simulink model "main_sim_adapt_Gref_SPPH"  (Simulink 7.2)
settings: Solver=ode2  SolverMode=SingleTasking  StartTime=0.0  StopTime=tsim_max  FixedStep=dtsim  RelTol=1e-3
StopFcn:
  | %mkplt
values from neighbouring files (symbols this model uses):
  assertion_time = inf    [setup_taem_sgs_al.m]
  cosA = cos(rwyAZ_rad)    [setup_taem_sgs_al.m]
  E_rwy = E_origin + (mod(( rwyLLA(2)/constants.r2d - lon_origin )+pi,2*pi)-pi) * constants.earth_radius * cos(lat_origin)    [setup_taem_sgs_al.m]
  eow_boundary = tmp_eow(ix(1))    [setup_taem_sgs_al.m]
  N_rwy = N_origin + (mod(( rwyLLA(1)/constants.r2d - lat_origin )+pi,2*pi)-pi) * constants.earth_radius    [setup_taem_sgs_al.m]
  sinA = sin(rwyAZ_rad)    [setup_taem_sgs_al.m]
  vel = 487.2512    [doit.m]
undefined symbols (not defined in the file or in its folder): accel_cmd, aero_surf_qbar_off, aero_surf_qbar_on, Alon, att_cmd_select, att_trim_IC, att_type, att_type_numbers, B1, bb_ellipsoid, bb_params, Blon, C, CA, chi_trim_IC, Clon, command_time, compute_all_rate_cols, compute_all_vel_cols, constants, da_trim_IC, dc_L2W_IC, de_trim_IC, DiscIntNeverNeededParam, dr_trim_IC, dtsim, DZkx, DZtheta, E_trim_IC, Ed_cmd, Ed_trim_IC, fc, flag_uad, full_surf_llim, full_surf_ulim, gain_set, gain_var_struct, gam_cmd_descent, gam_cmd_preflare, gamdot_cmd_descent, gamdot_cmd_flare, gamdot_cmd_preflare, gamma_trim_IC, Gamtheta, Gamx, h_trim_IC, hd_cmd, hd_trim_IC, ideal_vel_Kb, in_exsig_vecin, in_exsig_vecout, invCB, Kb, Kxhat0, Kxnom, Kxstar, lonxm0, MACH, MACH_att_fb, MACH_att_int_IC ... (+77)
libraries: simulink x36, utility_lib x36, mach_lib x24, model_lib x15, simulink_need_slupdate x8, models x6
(part 2 of 7)

== system main_sim_adapt_Gref_SPPH/claw_main/set scoped signals ==
  signal_bus : Inport  OutDataType=sfix(16)  OutScaling=2^0
  Bus Selector3 : BusSelector  OutputSignals=y_meas.h_geodetic,mode_sw.use_held_aero_obac_sw,y_meas.w_est,y_meas.NEh_dot,mode_sw.att_type,u_est,engines
  Gain1 : Gain  Orientation=left  Gain=use_variable_mass  ParameterDataType=sfix(16)  ParameterScaling=2^0  OutDataType=sfix(16)  OutScaling=2^0
  hold altitude : model_lib/hold input  SystemSampleTime=-1
  mass : DiscreteIntegrator  gainval=1  InitialCondition=MACH_mass_IC  SampleTime=-1  OutDataType=sfix(16)  OutScaling=2^0  ICPrevOutput=DiscIntNeverNeededParam  ICPrevScaledInput=DiscIntNeverNeededParam
  set scoped bus : model_lib/set scoped bus  SystemSampleTime=-1  vehicle_params=obac_params
  set scoped signals : model_lib/set scoped signals  SystemSampleTime=-1
  scoped_bus : Outport  OutDataType=sfix(16)  OutScaling=2^0
  wires:
  signal_bus/1 -> Bus Selector3/1
  Gain1/1 -> mass/1
  Bus Selector3/1 -> hold altitude/1  "<h_geodetic>"
  set scoped bus/2 -> Gain1/1
  set scoped bus/1 -> set scoped signals/1, scoped_bus/1
  mass/1 -> set scoped bus/7
  Bus Selector3/2 -> hold altitude/2  "<use_held_aero_obac_sw>"
  hold altitude/1 -> set scoped bus/1
  Bus Selector3/3 -> set scoped bus/2  "<w_est>"
  Bus Selector3/4 -> set scoped bus/3  "<NEh_dot>"
  Bus Selector3/5 -> set scoped bus/4  "<att_type>"
  Bus Selector3/6 -> set scoped bus/5  "<u_est>"
  Bus Selector3/7 -> set scoped bus/6  "<engines>"

== system main_sim_adapt_Gref_SPPH/claw_main/state est ==
  u_old : Inport  OutDataType=sfix(16)  OutScaling=2^0
  sensors : Inport  Port=2  OutDataType=sfix(16)  OutScaling=2^0
  signal_bus : Inport  Port=3  OutDataType=sfix(16)  OutScaling=2^0
  Bus Creator : BusCreator  Inputs=12
  Bus Creator1 : BusCreator  Inputs=6
  Bus Selector : BusSelector  OutputSignals=mode_sw.reset_pos_sw,mode_sw.nav_enable_sw,mode_sw.wind_est_sw
  Bus Selector1 : BusSelector  OutputSignals=nav_ok,pqr,NED_dot,latlonh,e
  Bus Selector2 : BusSelector  OutputSignals=aero_env.Mach,aero_env.vel,aero_env.alpha,aero_env.beta,aero_env.uvw_rw,aero_env.qbar
  Bus Selector3 : BusSelector  OutputSignals=u_meas,seeker,accels_cg
  Logical Operator : Logic  AllPortsSameDT=off  OutDataTypeMode=boolean  OutDataTypeStr=boolean
  beta_360 : Fcn  Expr=atan2(u(2),u(1))
  cl model : models/gtm-obac  SystemSampleTime=-1
  process inputs : Subsystem
  process sensors : Subsystem
  wind estimator : Subsystem
  y_meas : Outport  OutDataType=sfix(16)  OutScaling=2^0
  x_est : Outport  Port=2  OutDataType=sfix(16)  OutScaling=2^0
  xdot_est : Outport  Port=3  OutDataType=sfix(16)  OutScaling=2^0
  u_est : Outport  Port=4  OutDataType=sfix(16)  OutScaling=2^0
  aero_env_est : Outport  Port=5  OutDataType=sfix(16)  OutScaling=2^0
  w_est_debug : Outport  Port=6  OutDataType=sfix(16)  OutScaling=2^0
  wires:
  sensors/1 -> Bus Selector3/1, process inputs/2(sensors), wind estimator/3(sensors), Bus Selector1/1
  wind estimator/1(w_est) -> cl model/3, Bus Creator/12  "w_est"
  process sensors/8(dircos) -> wind estimator/1(dircos), Bus Creator/11  "dircos"
  cl model/1 -> xdot_est/1
  process sensors/9(x_est) -> cl model/1, wind estimator/2(x), x_est/1
  signal_bus/1 -> Bus Selector/1
  Bus Selector/1 -> process sensors/1(reset_pos)  "<reset_pos_sw>"
  Bus Selector/3 -> wind estimator/5(wind_est_sw)  "<wind_est_sw>"
  process inputs/1(u_est) -> u_est/1, cl model/2, wind estimator/4(u)
  Bus Selector1/2 -> process sensors/3(pqr)  "<pqr>"
  Bus Selector1/3 -> process sensors/4(NED_dot)  "<NED_dot>"
  Bus Selector1/4 -> process sensors/5(latlonh)  "<latlonh>"
  Bus Selector1/5 -> process sensors/6(e)  "<e>"
  process sensors/2(h_geodetic) -> Bus Creator/5  "h_geodetic"
  process sensors/3(NEh_nav) -> Bus Creator/6  "NEh_nav"
  process sensors/4(nav_valid) -> Bus Creator/7  "nav_valid"
  process sensors/5(NEh_dot) -> Bus Creator/8  "NEh_dot"
  process sensors/1(vehicle_origin) -> Bus Creator/4  "vehicle_origin"
  process sensors/7(cvc_origin) -> Bus Creator/10  "cvc_origin"
  u_old/1 -> process inputs/1(u_old)
  wind estimator/2(w_est_debug) -> w_est_debug/1
  cl model/2 -> Bus Selector2/1
  Bus Creator1/1 -> aero_env_est/1
  Logical Operator/1 -> process sensors/2(nav_ok)
  Bus Selector1/1 -> Logical Operator/2  "<nav_ok>"
  Bus Selector/2 -> Logical Operator/1  "<nav_enable_sw>"
  Bus Selector2/5 -> beta_360/1  "<uvw_rw>"
  process sensors/6(dc_fltpath) -> Bus Creator/9  "dc_fltpath"
  beta_360/1 -> Bus Creator1/5  "beta_360"
  Bus Selector2/1 -> Bus Creator1/1  "<Mach>"
  Bus Selector2/2 -> Bus Creator1/2  "<vel>"
  Bus Selector2/3 -> Bus Creator1/3  "<alpha>"
  Bus Selector2/4 -> Bus Creator1/4  "<beta>"
  Bus Selector2/6 -> Bus Creator1/6  "<qbar>"
  Bus Selector3/1 -> Bus Creator/1  "<u_meas>"
  Bus Selector3/2 -> Bus Creator/2  "<seeker>"
  Bus Selector3/3 -> Bus Creator/3  "<accels_cg>"
  Bus Creator/1 -> y_meas/1

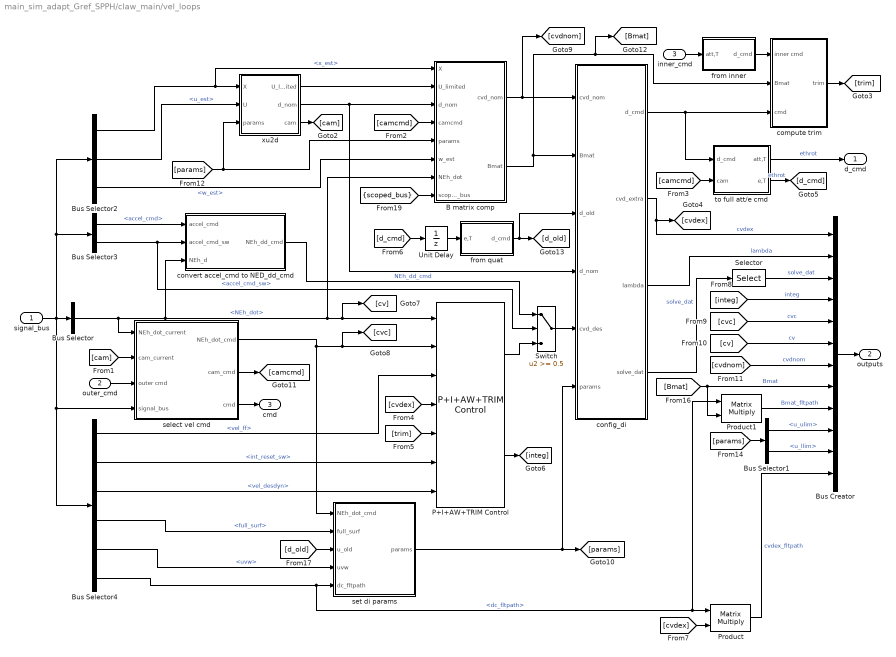
== system main_sim_adapt_Gref_SPPH/claw_main/vel_loops ==
  signal_bus : Inport  OutDataType=sfix(16)  OutScaling=2^0
  outer_cmd : Inport  Port=2  OutDataType=sfix(16)  OutScaling=2^0
  inner_cmd : Inport  Port=3  OutDataType=sfix(16)  OutScaling=2^0
  B matrix comp : Subsystem
  Bus Creator : BusCreator  Inputs=12
  Bus Selector : BusSelector  OutputSignals=y_meas.NEh_dot
  Bus Selector1 : BusSelector  OutputSignals=u_ulim,u_llim
  Bus Selector2 : BusSelector  OutputSignals=x_est,u_est,y_meas.w_est
  Bus Selector3 : BusSelector  OutputSignals=control_params.accel_cmd,control_params.accel_cmd_sw
  Bus Selector4 : BusSelector  OutputSignals=feed_forward.vel_ff,mode_sw.int_reset_sw,control_params.vel_desdyn,full_surf,x_est.uvw,y_meas.dc_fltpath
  P+I+AW+TRIM Control : mach_lib/P+I+AW+TRIM Control  SystemSampleTime=-1
  Product : Product  Multiplication=Matrix(*)  OutDataType=sfix(16)  OutScaling=2^0  RndMeth=Zero
  Product1 : Product  Multiplication=Matrix(*)  OutDataType=sfix(16)  OutScaling=2^0  RndMeth=Zero
  Selector : Selector  NumberOfDimensions=2  InputPortWidth=MACH.num_u  IndexOptions=Index vector (dialog),Index vector (dialog)  Indices=1:9,1:2  OutputSizes=1
  Switch : Switch  Threshold=0.5
  Unit Delay : UnitDelay  X0=MACH_vel_uold_IC  SampleTime=-1
  compute trim : Subsystem
  config_di : Subsystem  BlockChoice=di_smn  mask{num_cv=MACH.vel_num_cv, num_u=MACH.vel_num_u, wght_cv_type=MACH.vel_wght_cv_type}
      link override di_smn/config_smn/smn_sfunc: sfunc_name=MACH.smn_sfunc_name
      link override di_smn/config_smn/smn_sfunc/S-Function: FunctionName=smn_sfunc_gam_mpass_epsposdef
      settings: AttributesFormatString=%<BlockChoice>  TemplateBlock=mach_lib/config_di  MemberBlocks=di_pseudoinv,di_smn
  convert accel_cmd to NED_dd_cmd : Subsystem  TreatAsAtomicUnit=on
  from inner : Subsystem
  from quat : Subsystem
  select vel cmd : Subsystem
  set di params : Subsystem
  to full att/e cmd : Subsystem
  xu2d : Subsystem
  d_cmd : Outport  OutDataType=sfix(16)  OutScaling=2^0
  outputs : Outport  Port=2  OutDataType=sfix(16)  OutScaling=2^0
  cmd : Outport  Port=3  OutDataType=sfix(16)  OutScaling=2^0
  wires:
  B matrix comp/2(Bmat) -> config_di/2(Bmat), compute trim/2(Bmat), [Bmat]
  to full att/e cmd/1(att,T) -> d_cmd/1  "ethrot"
  config_di/1(d_cmd) -> compute trim/3(cmd), to full att/e cmd/1(d_cmd)
  P+I+AW+TRIM Control/2 -> [integ]
  xu2d/2(d_nom) -> config_di/4(d_nom), B matrix comp/3(d_nom)
  Bus Selector/1 -> convert accel_cmd to NED_dd_cmd/3(NEh_d), B matrix comp/7(NEh_dot), P+I+AW+TRIM Control/1, [cv], select vel cmd/1(NEh_dot_current)  "<NEh_dot>"
  xu2d/3(cam) -> [cam]
  [cam] -> select vel cmd/2(cam_current)
  compute trim/1(trim) -> [trim]
  inner_cmd/1 -> from inner/1(att,T)
  from inner/1(d_cmd) -> compute trim/1(inner cmd)
  [camcmd] -> to full att/e cmd/2(cam)
  Bus Selector2/3 -> B matrix comp/6(w_est)  "<w_est>"
  [d_cmd] -> Unit Delay/1
  Unit Delay/1 -> from quat/1(e,T)
  set di params/1(params) -> [params], config_di/6(params)
  [params] -> xu2d/3(params), B matrix comp/5(params)
  xu2d/1(U_limited) -> B matrix comp/2(U_limited)
  [integ] -> Bus Creator/4  "integ"
  [cvc] -> Bus Creator/5  "cvc"
  [cv] -> Bus Creator/6  "cv"
  [cvdnom] -> Bus Creator/7  "cvdnom"
  [trim] -> P+I+AW+TRIM Control/5
  [cvdex] -> P+I+AW+TRIM Control/4
  Bus Selector4/2 -> P+I+AW+TRIM Control/6  "<int_reset_sw>"
  Bus Selector4/1 -> P+I+AW+TRIM Control/3  "<vel_ff>"
  B matrix comp/1(cvd_nom) -> [cvdnom], config_di/1(cvd_nom)
  [Bmat] -> Product1/2, Bus Creator/8  "Bmat"
  config_di/2(cvd_extra) -> [cvdex], Bus Creator/1  "cvdex"
  from quat/1(d_cmd) -> [d_old], config_di/3(d_old)
  Bus Selector4/4 -> set di params/2(full_surf)  "<full_surf>"
  Product/1 -> Bus Creator/12  "cvdex_fltpath"
  [params] -> Bus Selector1/1
  Bus Selector1/1 -> Bus Creator/10  "<u_ulim>"
  Bus Selector1/2 -> Bus Creator/11  "<u_llim>"
  [d_old] -> set di params/3(u_old)
  Bus Selector4/5 -> set di params/4(uvw)  "<uvw>"
  config_di/3(lambda) -> Bus Creator/2  "lambda"
  config_di/4(solve_dat) -> Selector/1  "solve_dat"
  [cvdex] -> Product/2
  Selector/1 -> Bus Creator/3  "solve_dat"
  [camcmd] -> B matrix comp/4(camcmd)
  [scoped_bus] -> B matrix comp/8(scoped_bus)
  Bus Selector2/1 -> xu2d/1(X), B matrix comp/1(X)  "<x_est>"
  Bus Selector2/2 -> xu2d/2(U)  "<u_est>"
  Bus Selector4/3 -> P+I+AW+TRIM Control/7  "<vel_desdyn>"
  Bus Selector3/1 -> convert accel_cmd to NED_dd_cmd/1(accel_cmd)  "<accel_cmd>"
  Switch/1 -> config_di/5(cvd_des)
  P+I+AW+TRIM Control/1 -> Switch/3
  convert accel_cmd to NED_dd_cmd/1(NEh_dd_cmd) -> Switch/1  "NEh_dd_cmd"
  signal_bus/1 -> Bus Selector/1, Bus Selector3/1, Bus Selector2/1, Bus Selector4/1, select vel cmd/4(signal_bus)
  Bus Selector3/2 -> convert accel_cmd to NED_dd_cmd/2(accel_cmd_sw), Switch/2  "<accel_cmd_sw>"
  Product1/1 -> Bus Creator/9  "Bmat_fltpath"
  Bus Selector4/6 -> Product/1, Product1/1, set di params/5(dc_fltpath)  "<dc_fltpath>"
  to full att/e cmd/2(e,T) -> [d_cmd]  "ethrot"
  outer_cmd/1 -> select vel cmd/3(outer cmd)
  select vel cmd/3(cmd) -> cmd/1
  select vel cmd/2(cam_cmd) -> [camcmd]
  select vel cmd/1(NEh_dot_cmd) -> set di params/1(NEh_dot_cmd), P+I+AW+TRIM Control/2, [cvc]
  Bus Creator/1 -> outputs/1

== system main_sim_adapt_Gref_SPPH/control input (modified)/Add Excitation ==
  In : Inport
  Bus Selector1 : BusSelector  OutputSignals=command
  Demux : Demux  Outputs=[1 1 1 1]
  Excitation  Signal : Subsystem
  Mux : Mux
  Rate Transition2 : RateTransition  OutPortSampleTime=MACH.dt
  Step : Step  SampleTime=MACH.dt
  Sum : Sum  Inputs=|++  OutDataType=sfix(16)  OutScaling=2^0
  Out : Outport
  wires:
  Bus Selector1/1 -> Demux/1  "<command>"
  Demux/1 -> Mux/1
  Demux/3 -> Mux/3
  Demux/2 -> Sum/1
  Sum/1 -> Mux/2
  Step/1 -> Excitation  Signal/Enable
  Excitation  Signal/1(exsig) -> Rate Transition2/1
  Rate Transition2/1 -> Sum/2
  Demux/4 -> Mux/4
  In/1 -> Bus Selector1/1
  Mux/1 -> Out/1

== system main_sim_adapt_Gref_SPPH/control input (modified)/control input ==
  Rate Transition1 : RateTransition  OutPortSampleTime=MACH.dt
  form control input : Subsystem  SystemSampleTime=MACH.dt
  generate commands : Subsystem
  control_input : Outport  OutDataType=sfix(16)  OutScaling=2^0
  wires:
  Rate Transition1/1 -> control_input/1
  form control input/1(control_input) -> Rate Transition1/1
  generate commands/1(cmd_bus) -> form control input/1(cmd_bus)

== system main_sim_adapt_Gref_SPPH/control input (modified)/ideal responses ==
  control_input : Inport  OutDataType=sfix(16)  OutScaling=2^0
      settings: BusObject=control_input_bus
  ideal att rate response : Subsystem
  ideal pos vel response : Subsystem
  wires:
  control_input/1 -> ideal att rate response/1(control_input), ideal pos vel response/1(control_input)

== system main_sim_adapt_Gref_SPPH/vehicle_model/a/c model ==
  u : Inport  OutDataType=sfix(16)  OutScaling=2^0
  integrate_state : Inport  Port=2  OutDataType=sfix(16)  OutScaling=2^0
  NED_wind : Inport  Port=3  OutDataType=sfix(16)  OutScaling=2^0
  Logical Operator : Logic  Operator=NOT  AllPortsSameDT=off  OutDataTypeMode=boolean  OutDataTypeStr=boolean
  Product : Product  OutDataType=sfix(16)  OutScaling=2^0  RndMeth=Zero
  e mag error feedback : model_lib/e mag error feedback  SystemSampleTime=-1
  vehicle model : models/gtm-trac  SystemSampleTime=-1  vehicle_params=trac_params
  vehicle state integrator : Integrator  ExternalReset=level  InitialCondition=x_trac_IC
  x : Outport  OutDataType=sfix(16)  OutScaling=2^0
  xdot : Outport  Port=2  OutDataType=sfix(16)  OutScaling=2^0
  y : Outport  Port=3  OutDataType=sfix(16)  OutScaling=2^0
  wires:
  u/1 -> vehicle model/2
  vehicle state integrator/1 -> x/1, vehicle model/1, e mag error feedback/1
  integrate_state/1 -> Logical Operator/1, Product/2
  Product/1 -> xdot/1, vehicle state integrator/1
  Logical Operator/1 -> vehicle state integrator/2
  NED_wind/1 -> vehicle model/3
  vehicle model/2 -> y/1
  e mag error feedback/1 -> Product/1
  vehicle model/1 -> e mag error feedback/2

== system main_sim_adapt_Gref_SPPH/vehicle_model/apply additional limits ==
  effector_limits_in : Inport  OutDataType=sfix(16)  OutScaling=2^0
  Bus Assignment : BusAssignment  AssignedSignals=u_ulim,u_llim
  Bus Selector : BusSelector  OutputSignals=u_ulim,u_llim
  throt out of fuel limits : model_lib/throt out of fuel limits  SystemSampleTime=-1
  effector_limits : Outport  OutDataType=sfix(16)  OutScaling=2^0
  wires:
  effector_limits_in/1 -> Bus Assignment/1, Bus Selector/1
  Bus Selector/1 -> throt out of fuel limits/1  "<u_ulim>"
  Bus Selector/2 -> throt out of fuel limits/2  "<u_llim>"
  Bus Assignment/1 -> effector_limits/1
  throt out of fuel limits/1 -> Bus Assignment/2
  throt out of fuel limits/2 -> Bus Assignment/3

== system main_sim_adapt_Gref_SPPH/vehicle_model/set scoped signals ==
  note: Note: att_type is not actually
      | used by the trac
  output_bus : Inport  OutDataType=sfix(16)  OutScaling=2^0
  Bus Selector1 : BusSelector  OutputSignals=x,use_held_aero_trac_sw,NED_wind,xdot,u_servo,engines
  Constant2 : Constant  Value=MACH.att_type  OutDataType=sfix(16)  OutScaling=2^0
  Gain1 : Gain  Orientation=left  Gain=use_variable_mass  ParameterDataType=sfix(16)  ParameterScaling=2^0  OutDataType=sfix(16)  OutScaling=2^0
  NEh_dot : Selector  InputPortWidth=trac_params.num_x  IndexOptions=Index vector (dialog)  Indices=MACH.NEh_idx  OutputSizes=1
  h : Selector  InputPortWidth=MACH.num_x  IndexOptions=Index vector (dialog)  Indices=MACH.NEh_idx(3)  OutputSizes=1
  hold altitude : model_lib/hold input  SystemSampleTime=-1
  mass integrator : Integrator  InitialCondition=trac_params.mass_IC
  set scoped bus : model_lib/set scoped bus  SystemSampleTime=-1  vehicle_params=trac_params
  set scoped signals : model_lib/set scoped signals  SystemSampleTime=-1
  scoped_bus : Outport  OutDataType=sfix(16)  OutScaling=2^0
  wires:
  Bus Selector1/1 -> h/1  "<x>"
  NEh_dot/1 -> set scoped bus/3
  Bus Selector1/3 -> set scoped bus/2  "<NED_wind>"
  Bus Selector1/5 -> set scoped bus/5  "<u_servo>"
  mass integrator/1 -> set scoped bus/7
  set scoped bus/2 -> Gain1/1
  Gain1/1 -> mass integrator/1
  hold altitude/1 -> set scoped bus/1
  h/1 -> hold altitude/1
  Bus Selector1/2 -> hold altitude/2  "<use_held_aero_trac_sw>"
  set scoped bus/1 -> set scoped signals/1, scoped_bus/1
  Constant2/1 -> set scoped bus/4
  Bus Selector1/4 -> NEh_dot/1  "<xdot>"
  output_bus/1 -> Bus Selector1/1
  Bus Selector1/6 -> set scoped bus/6  "<engines>"

== system main_sim_adapt_Gref_SPPH/vehicle_model/target/seeker model ==
  output_bus : Inport  OutDataType=sfix(16)  OutScaling=2^0
  Bus Selector : BusSelector  OutputSignals=x,xdot
  Bus Selector1 : BusSelector  OutputSignals=LOS_rate,aux_info.azimuth,aux_info.elevation,aux_info.Rground,aux_info.Rslant
  Constant2 : Constant  Value=target_vel_IC  OutDataType=sfix(16)  OutScaling=2^0
  NEh : Selector  InputPortWidth=MACH.num_x  IndexOptions=Index vector (dialog)  Indices=MACH.NEh_idx  OutputSizes=1
  NEh_dot : Selector  InputPortWidth=MACH.num_x  IndexOptions=Index vector (dialog)  Indices=MACH.NEh_idx  OutputSizes=1
  seeker model : Subsystem
  seeker scope : Scope  NumInputPorts=5
      settings: YMin=-1.75~-3.5~-1.75~0~0  YMax=0.25~0.5~0~450000~550000
  target position integrator : Integrator  InitialCondition=target_pos_IC
  seeker : Outport  OutDataType=sfix(16)  OutScaling=2^0
  wires:
  Constant2/1 -> target position integrator/1, seeker model/2(NEh_d_target)
  target position integrator/1 -> seeker model/1(NEh_target)
  NEh/1 -> seeker model/3(NEh)
  NEh_dot/1 -> seeker model/4(NEh_d)
  seeker model/1(seeker) -> seeker/1, Bus Selector1/1
  output_bus/1 -> Bus Selector/1
  Bus Selector/1 -> NEh/1  "<x>"
  Bus Selector/2 -> NEh_dot/1  "<xdot>"
  Bus Selector1/2 -> seeker scope/2  "<azimuth>"
  Bus Selector1/3 -> seeker scope/3  "<elevation>"
  Bus Selector1/4 -> seeker scope/4  "<Rground>"
  Bus Selector1/5 -> seeker scope/5  "<Rslant>"
  Bus Selector1/1 -> seeker scope/1  "<LOS_rate>"

== system main_sim_adapt_Gref_SPPH/claw_main/att_loops/P+I+AW+TRIM Control ==
  cv : Inport  OutDataType=sfix(16)  OutScaling=2^0
  cv cmd : Inport  Port=2  OutDataType=sfix(16)  OutScaling=2^0
  cvd ff : Inport  Port=3  OutDataType=sfix(16)  OutScaling=2^0
  cvdot extra : Inport  Port=4  OutDataType=sfix(16)  OutScaling=2^0
  trim : Inport  Port=5  OutDataType=sfix(16)  OutScaling=2^0
  reset : Inport  Port=6  OutDataType=sfix(16)  OutScaling=2^0
  x0 : Inport  Port=7  OutDataType=sfix(16)  OutScaling=2^0
  Dot Product2 : simulink/Math Operations/Dot Product  InputSameDT=on  OutDataType=sfix(16)  OutScaling=2^-10  DoSatur=off
  P+I+AW+TRIM Control : mach_lib/P+I+AW+TRIM Control  SystemSampleTime=-1
  Product2 : Product  OutDataType=sfix(16)  OutScaling=2^0  SaturateOnIntegerOverflow=on  InputSameDT=on  OutDataTypeStr=Inherit: Same as first input
  Sum : Sum  Inputs=-+|  OutDataType=sfix(16)  OutScaling=2^0  SaturateOnIntegerOverflow=on
  Unit Delay1 : UnitDelay  SampleTime=-1
  fe : Gain  Gain=MACH.att_fe  ParameterDataType=sfix(16)  ParameterScaling=2^0  OutDataType=sfix(16)  OutScaling=2^0  SaturateOnIntegerOverflow=on  OutDataTypeStr=Inherit: Same as input  ParamDataTypeStr=Inherit: Same as input
  cvdot des : Outport  OutDataType=sfix(16)  OutScaling=2^0
  int state : Outport  Port=2  OutDataType=sfix(16)  OutScaling=2^0
  wires:
  cvd ff/1 -> P+I+AW+TRIM Control/3
  cvdot extra/1 -> P+I+AW+TRIM Control/4
  Sum/1 -> P+I+AW+TRIM Control/5
  reset/1 -> P+I+AW+TRIM Control/6
  x0/1 -> P+I+AW+TRIM Control/7
  fe/1 -> Sum/1
  trim/1 -> Sum/2
  Product2/1 -> fe/1
  Unit Delay1/1 -> Dot Product2/2
  Dot Product2/1 -> Product2/2
  P+I+AW+TRIM Control/2 -> int state/1
  P+I+AW+TRIM Control/1 -> Unit Delay1/1, cvdot des/1
  cv cmd/1 -> P+I+AW+TRIM Control/2
  cv/1 -> Product2/1, Dot Product2/1, P+I+AW+TRIM Control/1

== system main_sim_adapt_Gref_SPPH/claw_main/att_loops/compute trim ==
  inner cmd : Inport  OutDataType=sfix(16)  OutScaling=2^0
  Bmat : Inport  Port=2  OutDataType=sfix(16)  OutScaling=2^0
  cmd : Inport  Port=3  OutDataType=sfix(16)  OutScaling=2^0
  Product : Product  Multiplication=Matrix(*)  OutDataType=sfix(16)  OutScaling=2^0  SaturateOnIntegerOverflow=on  OutDataTypeStr=Inherit: Same as first input
  Sum1 : Sum  Inputs=|+-  OutDataType=sfix(16)  OutScaling=2^0  SaturateOnIntegerOverflow=on
  trim : Outport  OutDataType=sfix(16)  OutScaling=2^0
  wires:
  Product/1 -> trim/1
  Bmat/1 -> Product/1
  Sum1/1 -> Product/2
  inner cmd/1 -> Sum1/1
  cmd/1 -> Sum1/2

== system main_sim_adapt_Gref_SPPH/claw_main/att_loops/dyn inv ==
  limit_pqr_cmd : Inport  OutDataType=sfix(16)  OutScaling=2^0
  uvw : Inport  Port=2  OutDataType=sfix(16)  OutScaling=2^0
  e nom : Inport  Port=3  OutDataType=sfix(16)  OutScaling=2^0
  e dot des : Inport  Port=4  OutDataType=sfix(16)  OutScaling=2^0
  Dot Product : simulink/Math Operations/Dot Product  InputSameDT=on  OutDataType=sfix(16)  OutScaling=2^-10  DoSatur=off
  Gain4 : Gain  Gain=0.5  ParameterDataType=sfix(16)  ParameterScaling=2^0  OutDataType=sfix(16)  OutScaling=2^0
  Limit rate cmd : Subsystem
  Product4 : Product  OutDataType=sfix(16)  OutScaling=2^0  SaturateOnIntegerOverflow=on  InputSameDT=on  OutDataTypeStr=Inherit: Same as first input
  Product5 : Product  Inputs=**  Multiplication=Matrix(*)  OutDataType=sfix(16)  OutScaling=2^0  SaturateOnIntegerOverflow=on  InputSameDT=on  OutDataTypeStr=Inherit: Same as first input
  Sum4 : Sum  Inputs=++-  OutDataType=sfix(16)  OutScaling=2^0  SaturateOnIntegerOverflow=on  InputSameDT=on  OutDataTypeStr=Inherit: Same as first input
  getedinv : utility_lib/getedinv  SystemSampleTime=-1
  Bmat : Outport  OutDataType=sfix(16)  OutScaling=2^0
  pqr : Outport  Port=2  OutDataType=sfix(16)  OutScaling=2^0
  cvdex : Outport  Port=3  OutDataType=sfix(16)  OutScaling=2^0
  wires:
  Limit rate cmd/1(pqr_limited) -> pqr/1, Product5/2
  Sum4/1 -> cvdex/1
  Product4/1 -> Sum4/2
  Product5/1 -> Sum4/1
  e dot des/1 -> Dot Product/2, Sum4/3, getedinv/1
  e nom/1 -> Product4/1, Dot Product/1, getedinv/2
  Dot Product/1 -> Product4/2
  getedinv/2 -> Gain4/1
  uvw/1 -> Limit rate cmd/2(uvw)
  getedinv/1 -> Limit rate cmd/3(pqr)
  limit_pqr_cmd/1 -> Limit rate cmd/1(limit_pqr_cmd)
  Gain4/1 -> Product5/1, Bmat/1

== system main_sim_adapt_Gref_SPPH/claw_main/att_loops/low pass filter ==
  e_cmd : Inport  OutDataType=sfix(16)  OutScaling=2^0
  signal_bus : Inport  Port=2  OutDataType=sfix(16)  OutScaling=2^0
  att_ff : Inport  Port=3  OutDataType=sfix(16)  OutScaling=2^0
  Bus Selector4 : BusSelector  OutputSignals=control_params.att_desdyn.kf,control_params.att_desdyn.kb
  Compare To Zero : simulink/Logic and Bit Operations/Compare To Zero  SystemSampleTime=-1  relop===  LogicOutDataTypeMode=boolean  ZeroCross=off
  Constant : Constant  Value=MACH_att_fb  OutDataType=sfix(16)  OutScaling=2^0
  Discrete-Time Integrator : DiscreteIntegrator  ExternalReset=sampled level  InitialConditionSource=external  SampleTime=-1  OutDataType=sfix(16)  OutScaling=2^0  ICPrevOutput=DiscIntNeverNeededParam  ICPrevScaledInput=DiscIntNeverNeededParam
  Product : Product  Inputs=3  OutDataType=sfix(16)  OutScaling=2^0  RndMeth=Zero
  Product1 : Product  OutDataType=sfix(16)  OutScaling=2^0  RndMeth=Zero
  Product2 : Product  OutDataType=sfix(16)  OutScaling=2^0  RndMeth=Zero
  Sum : Sum  Inputs=|+-  OutDataType=sfix(16)  OutScaling=2^0
  Sum1 : Sum  Inputs=++|  OutDataType=sfix(16)  OutScaling=2^0
  cv cmd : Outport  OutDataType=sfix(16)  OutScaling=2^0
  cvd ff : Outport  Port=2  OutDataType=sfix(16)  OutScaling=2^0
  wires:
  Product/1 -> Sum1/2
  e_cmd/1 -> Sum/1, Discrete-Time Integrator/3
  Sum/1 -> Product/3
  Sum1/1 -> Discrete-Time Integrator/1, cvd ff/1
  Discrete-Time Integrator/1 -> Sum/2, cv cmd/1
  signal_bus/1 -> Bus Selector4/1
  att_ff/1 -> Product1/1
  Product1/1 -> Sum1/1
  Compare To Zero/1 -> Discrete-Time Integrator/2
  Bus Selector4/2 -> Product/2  "<kb>"
  Product2/1 -> Product/1, Compare To Zero/1
  Bus Selector4/1 -> Product2/2, Product1/2  "<kf>"
  Constant/1 -> Product2/1

== system main_sim_adapt_Gref_SPPH/claw_main/att_loops/select att cmd ==
  e_current : Inport  OutDataType=sfix(16)  OutScaling=2^0
  throt_current : Inport  Port=2  OutDataType=sfix(16)  OutScaling=2^0
  outer cmd : Inport  Port=3  OutDataType=sfix(16)  OutScaling=2^0
  signal_bus : Inport  Port=4  OutDataType=sfix(16)  OutScaling=2^0
  Bus Selector1 : BusSelector  OutputSignals=cmd_bus.select_cmd.att
  Compare To Zero : simulink/Logic and Bit Operations/Compare To Zero  SystemSampleTime=-1  relop===  LogicOutDataTypeMode=boolean  ZeroCross=off
  Demux : Demux  Outputs=[ 4 1 ]
  Demux1 : Demux  Outputs=[ 3 MACH.num_u_throt ]
  Demux2 : Demux  Outputs=[ 1 3 ]
  Mux1 : Mux  Inputs=2
  Switch : Switch  Threshold=0.5
  Unit Delay2 : UnitDelay  X0=MACH_throttle_IC  SampleTime=-1
  att2e_ref : utility_lib/att2e_ref  SystemSampleTime=-1
  e2att : utility_lib/e2att  SystemSampleTime=-1
  get direct cmd : Subsystem
  switch att cmd : MultiPortSwitch  zeroidx=on  SaturateOnIntegerOverflow=on
  switch throt cmd : MultiPortSwitch  zeroidx=on  SaturateOnIntegerOverflow=on
  e_cmd : Outport  OutDataType=sfix(16)  OutScaling=2^0
  throt_cmd : Outport  Port=2  OutDataType=sfix(16)  OutScaling=2^0
  cmd : Outport  Port=3  OutDataType=sfix(16)  OutScaling=2^0
  wires:
  switch att cmd/1 -> att2e_ref/1, Mux1/1
  Bus Selector1/1 -> Demux/1  "<att>"
  get direct cmd/2(throt) -> switch throt cmd/3
  throt_current/1 -> Unit Delay2/1
  Demux/2 -> switch throt cmd/1
  outer cmd/1 -> Demux1/1
  Demux1/2 -> switch throt cmd/4
  switch throt cmd/1 -> throt_cmd/1, Mux1/2
  signal_bus/1 -> get direct cmd/1(signal_bus), Bus Selector1/1
  Demux/1 -> Demux2/1
  e_current/1 -> e2att/1, Switch/1, att2e_ref/2
  Unit Delay2/1 -> switch throt cmd/2
  get direct cmd/1(att) -> switch att cmd/3
  e2att/1 -> switch att cmd/2
  Demux1/1 -> switch att cmd/4
  att2e_ref/1 -> Switch/3
  Switch/1 -> e_cmd/1
  Demux2/1 -> Compare To Zero/1
  Demux2/2 -> switch att cmd/1
  Compare To Zero/1 -> Switch/2
  Mux1/1 -> cmd/1

== system main_sim_adapt_Gref_SPPH/claw_main/grab ExportedGlobal/grab cv variables ==
  In1 : Inport  OutDataType=sfix(16)  OutScaling=2^0
  Bus Selector6 : BusSelector  OutputSignals=rate.cv,att.cv,vel.cv,pos.cv
  Demux1 : Demux  Outputs=3
  Demux2 : Demux
  Demux3 : Demux  Outputs=3
  Demux4 : Demux  Outputs=3
  Mux : Mux  Inputs=13
  Subsystem : Subsystem  TreatAsAtomicUnit=on
      settings: RTWSystemCode=Inline
  Out1 : Outport  OutDataType=sfix(16)  OutScaling=2^0
  wires:
  Subsystem/1(Out1) -> Mux/1  "CLAW_p_cv"
  Subsystem/2(Out2) -> Mux/2  "CLAW_q_cv"
  Subsystem/3(Out3) -> Mux/3  "CLAW_r_cv"
  Subsystem/4(Out4) -> Mux/4  "CLAW_e0_cv"
  Subsystem/5(Out5) -> Mux/5  "CLAW_e1_cv"
  Subsystem/6(Out6) -> Mux/6  "CLAW_e2_cv"
  Subsystem/8(Out8) -> Mux/8  "CLAW_Ndot_cv"
  Subsystem/9(Out9) -> Mux/9  "CLAW_Edot_cv"
  Subsystem/10(Out10) -> Mux/10  "CLAW_hdot_cv"
  Subsystem/11(Out11) -> Mux/11  "CLAW_N_cv"
  Subsystem/12(Out12) -> Mux/12  "CLAW_E_cv"
  Subsystem/13(Out13) -> Mux/13  "CLAW_h_cv"
  Subsystem/7(Out7) -> Mux/7  "CLAW_e3_cv"
  In1/1 -> Bus Selector6/1
  Mux/1 -> Out1/1
  Demux1/1 -> Subsystem/1(In1)
  Demux1/2 -> Subsystem/2(In2)
  Demux1/3 -> Subsystem/3(In3)
  Demux2/1 -> Subsystem/4(In4)
  Demux2/2 -> Subsystem/5(In5)
  Demux2/3 -> Subsystem/6(In6)
  Demux2/4 -> Subsystem/7(In7)
  Demux3/1 -> Subsystem/8(In8)
  Demux3/2 -> Subsystem/9(In9)
  Demux3/3 -> Subsystem/10(In10)
  Demux4/1 -> Subsystem/11(In11)
  Demux4/2 -> Subsystem/12(In12)
  Demux4/3 -> Subsystem/13(In13)
  Bus Selector6/1 -> Demux1/1  "<cv>"
  Bus Selector6/2 -> Demux2/1  "<cv>"
  Bus Selector6/3 -> Demux3/1  "<cv>"
  Bus Selector6/4 -> Demux4/1  "<cv>"

== system main_sim_adapt_Gref_SPPH/claw_main/grab ExportedGlobal/grab cvcmd variables ==
  In1 : Inport  OutDataType=sfix(16)  OutScaling=2^0
  Bus Selector5 : BusSelector  OutputSignals=rate.cvc,att.cvc,vel.cvc,pos.cvc
  Demux1 : Demux  Outputs=3
  Demux2 : Demux
  Demux3 : Demux  Outputs=3
  Demux4 : Demux  Outputs=3
  Mux : Mux  Inputs=13
  Subsystem : Subsystem  TreatAsAtomicUnit=on
      settings: RTWSystemCode=Inline
  Out1 : Outport  OutDataType=sfix(16)  OutScaling=2^0
  wires:
  Subsystem/1(Out1) -> Mux/1  "CLAW_p_cvcmd"
  Subsystem/2(Out2) -> Mux/2  "CLAW_q_cvcmd"
  Subsystem/3(Out3) -> Mux/3  "CLAW_r_cvcmd"
  Subsystem/4(Out4) -> Mux/4  "CLAW_e0_cvcmd"
  Subsystem/5(Out5) -> Mux/5  "CLAW_e1_cvcmd"
  Subsystem/6(Out6) -> Mux/6  "CLAW_e2_cvcmd"
  Subsystem/8(Out8) -> Mux/8  "CLAW_Ndot_cvcmd"
  Subsystem/9(Out9) -> Mux/9  "CLAW_Edot_cvcmd"
  Subsystem/10(Out10) -> Mux/10  "CLAW_hdot_cvcmd"
  Subsystem/11(Out11) -> Mux/11  "CLAW_N_cvcmd"
  Subsystem/12(Out12) -> Mux/12  "CLAW_E_cvcmd"
  Subsystem/13(Out13) -> Mux/13  "CLAW_h_cvcmd"
  Subsystem/7(Out7) -> Mux/7  "CLAW_e3_cvcmd"
  In1/1 -> Bus Selector5/1
  Mux/1 -> Out1/1
  Demux1/1 -> Subsystem/1(In1)
  Demux1/2 -> Subsystem/2(In2)
  Demux1/3 -> Subsystem/3(In3)
  Demux2/1 -> Subsystem/4(In4)
  Demux2/2 -> Subsystem/5(In5)
  Demux2/3 -> Subsystem/6(In6)
  Demux2/4 -> Subsystem/7(In7)
  Demux3/1 -> Subsystem/8(In8)
  Demux3/2 -> Subsystem/9(In9)
  Demux3/3 -> Subsystem/10(In10)
  Demux4/1 -> Subsystem/11(In11)
  Demux4/2 -> Subsystem/12(In12)
  Demux4/3 -> Subsystem/13(In13)
  Bus Selector5/4 -> Demux4/1  "<cvc>"
  Bus Selector5/2 -> Demux2/1  "<cvc>"
  Bus Selector5/1 -> Demux1/1  "<cvc>"
  Bus Selector5/3 -> Demux3/1  "<cvc>"

== system main_sim_adapt_Gref_SPPH/claw_main/grab ExportedGlobal/grab cvdex variables ==
  In1 : Inport  OutDataType=sfix(16)  OutScaling=2^0
  Bus Selector3 : BusSelector  OutputSignals=rate.cvdex,att.cvdex,vel.cvdex,pos.cvdex
  Demux1 : Demux  Outputs=3
  Demux2 : Demux
  Demux3 : Demux  Outputs=3
  Demux4 : Demux  Outputs=3
  Mux : Mux  Inputs=13
  Subsystem : Subsystem  TreatAsAtomicUnit=on
      settings: RTWSystemCode=Inline
  Out1 : Outport  OutDataType=sfix(16)  OutScaling=2^0
  wires:
  Subsystem/1(Out1) -> Mux/1  "CLAW_p_cvdex"
  Subsystem/2(Out2) -> Mux/2  "CLAW_q_cvdex"
  Subsystem/3(Out3) -> Mux/3  "CLAW_r_cvdex"
  Subsystem/4(Out4) -> Mux/4  "CLAW_e0_cvdex"
  Subsystem/5(Out5) -> Mux/5  "CLAW_e1_cvdex"
  Subsystem/6(Out6) -> Mux/6  "CLAW_e2_cvdex"
  Subsystem/8(Out8) -> Mux/8  "CLAW_Ndot_cvdex"
  Subsystem/9(Out9) -> Mux/9  "CLAW_Edot_cvdex"
  Subsystem/10(Out10) -> Mux/10  "CLAW_hdot_cvdex"
  Subsystem/11(Out11) -> Mux/11  "CLAW_N_cvdex"
  Subsystem/12(Out12) -> Mux/12  "CLAW_E_cvdex"
  Subsystem/13(Out13) -> Mux/13  "CLAW_h_cvdex"
  Subsystem/7(Out7) -> Mux/7  "CLAW_e3_cvdex"
  Demux1/1 -> Subsystem/1(In1)
  Demux1/2 -> Subsystem/2(In2)
  Demux1/3 -> Subsystem/3(In3)
  Demux2/1 -> Subsystem/4(In4)
  Demux2/2 -> Subsystem/5(In5)
  Demux2/3 -> Subsystem/6(In6)
  Demux2/4 -> Subsystem/7(In7)
  Demux3/1 -> Subsystem/8(In8)
  Demux3/2 -> Subsystem/9(In9)
  Demux3/3 -> Subsystem/10(In10)
  Demux4/1 -> Subsystem/11(In11)
  Demux4/2 -> Subsystem/12(In12)
  Demux4/3 -> Subsystem/13(In13)
  Mux/1 -> Out1/1
  In1/1 -> Bus Selector3/1
  Bus Selector3/4 -> Demux4/1  "<cvdex>"
  Bus Selector3/3 -> Demux3/1  "<cvdex>"
  Bus Selector3/2 -> Demux2/1  "<cvdex>"
  Bus Selector3/1 -> Demux1/1  "<cvdex>"

== system main_sim_adapt_Gref_SPPH/claw_main/grab ExportedGlobal/grab integrator variables ==
  In1 : Inport  OutDataType=sfix(16)  OutScaling=2^0
  Bus Selector4 : BusSelector  OutputSignals=rate.integ,att.integ,vel.integ,pos.integ
  Demux1 : Demux  Outputs=3
  Demux2 : Demux
  Demux3 : Demux  Outputs=3
  Demux4 : Demux  Outputs=3
  Mux : Mux  Inputs=13
  Subsystem : Subsystem  TreatAsAtomicUnit=on
      settings: RTWSystemCode=Inline
  Out1 : Outport  OutDataType=sfix(16)  OutScaling=2^0
  wires:
  Subsystem/1(Out1) -> Mux/1  "CLAW_p_int"
  Subsystem/2(Out2) -> Mux/2  "CLAW_q_int"
  Subsystem/3(Out3) -> Mux/3  "CLAW_r_int"
  Subsystem/4(Out4) -> Mux/4  "CLAW_e0_int"
  Subsystem/5(Out5) -> Mux/5  "CLAW_e1_int"
  Subsystem/6(Out6) -> Mux/6  "CLAW_e2_int"
  Subsystem/8(Out8) -> Mux/8  "CLAW_Ndot_int"
  Subsystem/9(Out9) -> Mux/9  "CLAW_Edot_int"
  Subsystem/10(Out10) -> Mux/10  "CLAW_hdot_int"
  Subsystem/11(Out11) -> Mux/11  "CLAW_N_int"
  Subsystem/12(Out12) -> Mux/12  "CLAW_E_int"
  Subsystem/13(Out13) -> Mux/13  "CLAW_h_int"
  Subsystem/7(Out7) -> Mux/7  "CLAW_e3_int"
  Mux/1 -> Out1/1
  Demux1/1 -> Subsystem/1(In1)
  Demux1/2 -> Subsystem/2(In2)
  Demux1/3 -> Subsystem/3(In3)
  Demux2/1 -> Subsystem/4(In4)
  Demux2/2 -> Subsystem/5(In5)
  Demux2/3 -> Subsystem/6(In6)
  Demux2/4 -> Subsystem/7(In7)
  Demux3/1 -> Subsystem/8(In8)
  Demux3/2 -> Subsystem/9(In9)
  Demux3/3 -> Subsystem/10(In10)
  Demux4/1 -> Subsystem/11(In11)
  Demux4/2 -> Subsystem/12(In12)
  Demux4/3 -> Subsystem/13(In13)
  In1/1 -> Bus Selector4/1
  Bus Selector4/4 -> Demux4/1  "<integ>"
  Bus Selector4/3 -> Demux3/1  "<integ>"
  Bus Selector4/2 -> Demux2/1  "<integ>"
  Bus Selector4/1 -> Demux1/1  "<integ>"

== system main_sim_adapt_Gref_SPPH/claw_main/grab ExportedGlobal/grab w_est variables ==
  In1 : Inport  OutDataType=sfix(16)  OutScaling=2^0
  Bus Selector12 : BusSelector  OutputSignals=w_est_debug.w_est
  Demux1 : Demux  Outputs=3
  Mux : Mux  Inputs=3
  Subsystem : Subsystem  TreatAsAtomicUnit=on
      settings: RTWSystemCode=Inline
  Out1 : Outport  OutDataType=sfix(16)  OutScaling=2^0
  wires:
  Subsystem/1(Out1) -> Mux/1  "CLAW_Nd_wind"
  Subsystem/2(Out2) -> Mux/2  "CLAW_Ed_wind"
  Subsystem/3(Out3) -> Mux/3  "CLAW_Dd_wind"
  Demux1/1 -> Subsystem/1(In1)
  Demux1/2 -> Subsystem/2(In2)
  Demux1/3 -> Subsystem/3(In3)
  Mux/1 -> Out1/1
  Bus Selector12/1 -> Demux1/1  "<w_est>"
  In1/1 -> Bus Selector12/1

== system main_sim_adapt_Gref_SPPH/claw_main/input processing/mode dependent stick processing ==
  command : Inport  OutDataType=sfix(16)  OutScaling=2^0
  signal_bus : Inport  Port=2  OutDataType=sfix(16)  OutScaling=2^0
  Bus Creator : BusCreator  Inputs=2
  Bus Selector1 : BusSelector  OutputSignals=control_params.accel_cmd_sw,mode_sw.CLAW_mode
  Bus Selector2 : BusSelector  OutputSignals=y_meas.NEh_dot,x_est
  att rate cmd : Subsystem
  att_type cmd : Subsystem
  feed forward : Subsystem
  llh cmd : Subsystem
  rampin vel_cmd : Subsystem
  set command selection switches : Subsystem
  table iv computation : Subsystem
  use table lookup pos cmds : Subsystem
  cmd_bus : Outport  OutDataType=sfix(16)  OutScaling=2^0
  feed_forward : Outport  Port=2  OutDataType=sfix(16)  OutScaling=2^0
  wires:
  Bus Selector1/2 -> set command selection switches/2(CLAW_mode), att rate cmd/1(mode), llh cmd/1(mode), rampin vel_cmd/1(mode), use table lookup pos cmds/1(mode), att_type cmd/1(mode)  "<CLAW_mode>"
  signal_bus/1 -> Bus Selector1/1, llh cmd/3(signal_bus), att rate cmd/3(signal_bus), Bus Selector2/1, att_type cmd/3(signal_bus), feed forward/2(signal_bus)
  llh cmd/1(command_out) -> att rate cmd/2(command_in)
  Bus Selector2/1 -> rampin vel_cmd/3(NEh_dot)  "<NEh_dot>"
  Bus Selector1/1 -> set command selection switches/1(accel_cmd_sw)  "<accel_cmd_sw>"
  set command selection switches/1(select_cmd) -> Bus Creator/1  "select_cmd"
  rampin vel_cmd/1(command_out) -> use table lookup pos cmds/2(command_in)
  Bus Creator/1 -> cmd_bus/1
  use table lookup pos cmds/1(command_out) -> Bus Creator/2  "autopilot_cmd"
  Bus Selector2/2 -> table iv computation/1(x_est)  "<x_est>"
  table iv computation/1(table_bus) -> use table lookup pos cmds/3(table_bus), feed forward/1(table_bus)
  feed forward/1(feed_forward) -> feed_forward/1
  command/1 -> llh cmd/2(command_in)
  att_type cmd/1(command_out) -> rampin vel_cmd/2(command_in)
  att rate cmd/1(command_out) -> att_type cmd/2(command_in)

== system main_sim_adapt_Gref_SPPH/claw_main/input processing/modify limits and apply to direct commands ==
  note: Currently, the limits for direct mode and throttle in att and rate modes
      | are the same as those used for automatic control.  May want to revisit this someday ...
  u_old : Inport  OutDataType=sfix(16)  OutScaling=2^0
  u_meas : Inport  Port=2  OutDataType=sfix(16)  OutScaling=2^0
  full_surf_in : Inport  Port=3  OutDataType=sfix(16)  OutScaling=2^0
  Bus Assignment : BusAssignment  AssignedSignals=full_surf_cmd
  Bus Selector2 : BusSelector  OutputSignals=full_surf_ulim,full_surf_llim,full_surf_urlim,full_surf_lrlim,full_surf_cmd
  MinMax : MinMax  Inputs=2  OutDataType=sfix(16)  OutScaling=2^0  SaturateOnIntegerOverflow=on  InputSameDT=on
  MinMax2 : MinMax  Function=max  Inputs=2  OutDataType=sfix(16)  OutScaling=2^0  SaturateOnIntegerOverflow=on  InputSameDT=on
  apply surface locking : Subsystem
  limit computation : mach_lib/limit computation  SystemSampleTime=-1
  rate limit limits : mach_lib/rate limit limits  SystemSampleTime=-1  ulim=MACH.u_ulim  llim=MACH.u_llim
  throt out of fuel limits : Subsystem
  full_surf : Outport  OutDataType=sfix(16)  OutScaling=2^0
  wires:
  Bus Selector2/3 -> rate limit limits/4, limit computation/4  "<full_surf_urlim>"
  Bus Selector2/4 -> rate limit limits/5, limit computation/5  "<full_surf_lrlim>"
  rate limit limits/1 -> limit computation/2
  rate limit limits/2 -> limit computation/3
  limit computation/2 -> MinMax2/1
  limit computation/1 -> MinMax/1
  MinMax2/1 -> MinMax/2
  u_old/1 -> rate limit limits/1, limit computation/1
  Bus Selector2/2 -> rate limit limits/3  "<full_surf_llim>"
  Bus Selector2/5 -> MinMax2/2  "<full_surf_cmd>"
  MinMax/1 -> Bus Assignment/2
  throt out of fuel limits/1(full_surf) -> Bus Selector2/1, Bus Assignment/1
  Bus Selector2/1 -> rate limit limits/2  "<full_surf_ulim>"
  Bus Assignment/1 -> full_surf/1
  u_meas/1 -> apply surface locking/1(u_meas)
  full_surf_in/1 -> apply surface locking/2(full_surf_in)
  apply surface locking/1(full_surf) -> throt out of fuel limits/1(full_surf_in)

== system main_sim_adapt_Gref_SPPH/claw_main/input processing/select att_type ==
  scoped_bus : Inport  OutDataType=sfix(16)  OutScaling=2^0
  mode_sw_in : Inport  Port=2  OutDataType=sfix(16)  OutScaling=2^0
  signal_bus : Inport  Port=3  OutDataType=sfix(16)  OutScaling=2^0
  Bus Assignment : BusAssignment  AssignedSignals=att_type
  Bus Selector : BusSelector  OutputSignals=qbar,abs_vel_rw,abs_cos_beta,abs_cos_theta,abs_cos_b,abs_cos_gamma_rw
  Bus Selector1 : BusSelector  OutputSignals=att_type
  Constant5 : Constant  Value=use_auto_att_type  OutDataType=sfix(16)  OutScaling=2^0
  Multiport Switch1 : MultiPortSwitch  Inputs=2  zeroidx=on
  Product : Product  OutDataType=sfix(16)  OutScaling=2^0  RndMeth=Zero
  add tiebreaker for current att_type : Subsystem
  att type input : Scope  NumInputPorts=6
      settings: YMin=1~0~0~0.1~5.55112e-017~5.55112e-017  YMax=4~900~5000~1~1~1  SaveName=att_type_input
  att type output : Scope  NumInputPorts=2
      settings: YMin=1~0  YMax=4~2.5  SaveName=att_type_output
  compute precond vars : Subsystem
  evaluate preconditions : Subsystem
  priority_weighting : Constant  Value=[0 1 1 0 2 0]  OutDataType=sfix(16)  OutScaling=2^0
  select best att_type : Subsystem
  mode_sw : Outport  OutDataType=sfix(16)  OutScaling=2^0
  wires:
  scoped_bus/1 -> compute precond vars/2(scoped_bus)
  mode_sw_in/1 -> Bus Selector1/1, Bus Assignment/1
  signal_bus/1 -> compute precond vars/1(signal_bus)
  Bus Selector1/1 -> Multiport Switch1/2  "<att_type>"
  Bus Assignment/1 -> mode_sw/1
  add tiebreaker for current att_type/1(priority_out) -> Product/1
  Product/1 -> select best att_type/1(vec), att type output/2  "att_type_availability"
  select best att_type/1(idx_max) -> att type output/1, Multiport Switch1/3, add tiebreaker for current att_type/1(att_type_selected)  "att_type_selected"
  evaluate preconditions/1(precond_satisfied) -> Product/2
  Multiport Switch1/1 -> Bus Assignment/2
  Constant5/1 -> Multiport Switch1/1
  priority_weighting/1 -> add tiebreaker for current att_type/2(priority_in)
  compute precond vars/1(precond_vars) -> Bus Selector/1, evaluate preconditions/1(precond_vars)
  Bus Selector/1 -> att type input/1  "<qbar>"
  Bus Selector/2 -> att type input/2  "<abs_vel_rw>"
  Bus Selector/3 -> att type input/3  "<abs_cos_beta>"
  Bus Selector/4 -> att type input/4  "<abs_cos_theta>"
  Bus Selector/5 -> att type input/5  "<abs_cos_b>"
  Bus Selector/6 -> att type input/6  "<abs_cos_gamma_rw>"

== system main_sim_adapt_Gref_SPPH/claw_main/input processing/set control parameters ==
  note: (Optionally) disable bb
      |  while we still have fuel
  signal_bus : Inport  OutDataType=sfix(16)  OutScaling=2^0
  full_surf : Inport  Port=2  OutDataType=sfix(16)  OutScaling=2^0
  Bus Creator1 : BusCreator  Inputs=10
  Bus Selector1 : BusSelector  OutputSignals=mode_sw.enable_bb_sw,mode_sw.gain_set_sw
  Bus Selector3 : BusSelector  OutputSignals=aero_env_est
  Constant : Constant  OutDataType=sfix(16)  OutScaling=2^0
  Constant1 : Constant  OutDataType=sfix(16)  OutScaling=2^0
  Logical Operator : Logic  Operator=NOT  AllPortsSameDT=off
  Logical Operator1 : Logic  Operator=NOT  AllPortsSameDT=off
  Logical Operator4 : Logic  AllPortsSameDT=off
  Logical Operator5 : Logic  Operator=OR  AllPortsSameDT=off
  accel submode setup : Subsystem
  modify MACH_att_Kf : Subsystem
  out of fuel : model_lib/out of fuel ?  SystemSampleTime=-1
  select gains : Subsystem
  set att desdyn params : Subsystem
  set pos desdyn params : Subsystem
  set rate desdyn params : Subsystem
  set rate di params : Subsystem
  set vel desdyn params : Subsystem
  control_params : Outport  OutDataType=sfix(16)  OutScaling=2^0
  wires:
  set pos desdyn params/1(params) -> Bus Creator1/6  "pos_desdyn"
  set vel desdyn params/1(params) -> Bus Creator1/7  "vel_desdyn"
  set att desdyn params/1(params) -> Bus Creator1/8  "att_desdyn"
  set rate desdyn params/1(params) -> Bus Creator1/9  "rate_desdyn"
  Bus Selector1/1 -> Logical Operator4/1  "<enable_bb_sw>"
  Logical Operator/1 -> Bus Creator1/3  "limit_pqr_cmd"
  Logical Operator4/1 -> select gains/1(enable_bb), Logical Operator/1, Bus Creator1/4  "enable_bb"
  select gains/2(gain_bus) -> set pos desdyn params/1(gain_bus), set vel desdyn params/1(gain_bus), set rate desdyn params/1(gain_bus), modify MACH_att_Kf/1(gain_bus_in)
  Bus Creator1/1 -> control_params/1
  select gains/1(gain_set) -> Bus Creator1/5  "gain_set"
  Constant/1 -> out of fuel/1
  out of fuel/1 -> Logical Operator1/1
  Logical Operator1/1 -> Logical Operator5/1
  Logical Operator5/1 -> Logical Operator4/2
  Constant1/1 -> Logical Operator5/2
  Bus Selector1/2 -> select gains/2(gain_set_in)  "<gain_set_sw>"
  accel submode setup/2(accel_cmd) -> Bus Creator1/2  "accel_cmd"
  accel submode setup/1(accel_cmd_sw) -> Bus Creator1/1  "accel_cmd_sw"
  signal_bus/1 -> accel submode setup/1(signal_bus), Bus Selector1/1, Bus Selector3/1, modify MACH_att_Kf/2(signal_bus)
  set rate di params/1(rate_params) -> Bus Creator1/10  "rate_params"
  Bus Selector3/1 -> set rate di params/2(aero_env_est)  "<aero_env_est>"
  full_surf/1 -> set rate di params/1(full_surf)
  modify MACH_att_Kf/1(gain_bus) -> set att desdyn params/1(gain_bus)

== system main_sim_adapt_Gref_SPPH/claw_main/pos_loops/compute trim ==
  inner cmd : Inport  OutDataType=sfix(16)  OutScaling=2^0
  cmd : Inport  Port=2  OutDataType=sfix(16)  OutScaling=2^0
  Sum1 : Sum  Inputs=|+-  OutDataType=sfix(16)  OutScaling=2^0  SaturateOnIntegerOverflow=on
  trim : Outport  OutDataType=sfix(16)  OutScaling=2^0
  wires:
  Sum1/1 -> trim/1
  inner cmd/1 -> Sum1/1
  cmd/1 -> Sum1/2

== system main_sim_adapt_Gref_SPPH/claw_main/pos_loops/limiter ==
  vel_inner_cmd : Inport  OutDataType=sfix(16)  OutScaling=2^0
  signal_bus : Inport  Port=2  OutDataType=sfix(16)  OutScaling=2^0
  cvd_des_in : Inport  Port=3  OutDataType=sfix(16)  OutScaling=2^0
  Bus Selector2 : BusSelector  OutputSignals=cmd_bus.select_cmd.vel,feed_forward.pos_ff,y_meas.dc_fltpath
  Compare To Constant : simulink/Logic and Bit Operations/Compare To Constant  SystemSampleTime=-1  relop=<  const=2  LogicOutDataTypeMode=boolean  ZeroCross=off
  Constant : Constant  Value=use_pos_fltpath_lim  OutDataType=sfix(16)  OutScaling=2^0
  Math Function : Math  Operator=transpose  OutDataType=sfix(16)  OutScaling=2^0  SaturateOnIntegerOverflow=on
  Product : Product  Multiplication=Matrix(*)  OutDataType=sfix(16)  OutScaling=2^0  RndMeth=Zero
  Product1 : Product  Multiplication=Matrix(*)  OutDataType=sfix(16)  OutScaling=2^0  RndMeth=Zero
  Saturation : Saturate  UpperLimit=MACH.pos_u_ulim  LowerLimit=MACH.pos_u_llim
  Saturation1 : Saturate  UpperLimit=MACH.pos_fltpath_u_ulim  LowerLimit=MACH.pos_fltpath_u_llim
  Selector1 : Selector  InputPortWidth=4  IndexOptions=Index vector (dialog)  Indices=[1 2 4]  OutputSizes=1
  Sum : Sum  Inputs=-+|  OutDataType=sfix(16)  OutScaling=2^0
  Sum1 : Sum  Inputs=++|  OutDataType=sfix(16)  OutScaling=2^0
  Sum2 : Sum  Inputs=+-|  OutDataType=sfix(16)  OutScaling=2^0  SaturateOnIntegerOverflow=on  InputSameDT=on  OutDataTypeStr=Inherit: Same as first input
  Switch : Switch  Threshold=0.5
  Switch1 : Switch  Threshold=0.5
  Unit Delay : UnitDelay  X0=MACH_vel_IC  SampleTime=MACH.dt
  cvd_des : Outport  OutDataType=sfix(16)  OutScaling=2^0
  cvd_extra : Outport  Port=2  OutDataType=sfix(16)  OutScaling=2^0
  wires:
  Switch1/1 -> Sum1/1, Sum/1
  Constant/1 -> Switch/2
  Saturation/1 -> Switch/3
  Switch/1 -> cvd_des/1, Sum2/1
  Sum1/1 -> Switch/1
  cvd_des_in/1 -> Sum/2, Saturation/1, Sum2/2
  Bus Selector2/3 -> Product/1, Math Function/1  "<dc_fltpath>"
  Sum/1 -> Product/2
  Product/1 -> Saturation1/1
  Saturation1/1 -> Product1/2
  Math Function/1 -> Product1/1
  Product1/1 -> Sum1/2
  Sum2/1 -> cvd_extra/1
  signal_bus/1 -> Bus Selector2/1
  Bus Selector2/1 -> Selector1/1  "<vel>"
  Bus Selector2/2 -> Switch1/3  "<pos_ff>"
  Compare To Constant/1 -> Switch1/2
  Selector1/1 -> Compare To Constant/1
  Unit Delay/1 -> Switch1/1
  vel_inner_cmd/1 -> Unit Delay/1

== system main_sim_adapt_Gref_SPPH/claw_main/pos_loops/select pos cmd ==
  NEh_current : Inport  OutDataType=sfix(16)  OutScaling=2^0
  outer cmd : Inport  Port=2  OutDataType=sfix(16)  OutScaling=2^0
  signal_bus : Inport  Port=3  OutDataType=sfix(16)  OutScaling=2^0
  Bus Selector : BusSelector  OutputSignals=cmd_bus.select_cmd.pos,cmd_bus.autopilot_cmd
  Demux3 : Demux  Outputs=[ 3 1 ]
  Ground : Ground
  Multiport Switch : MultiPortSwitch  zeroidx=on  SaturateOnIntegerOverflow=on
  Mux1 : Mux  Inputs=2
  Selector2 : Selector  InputPortWidth=4  IndexOptions=Index vector (dialog)  Indices=[1 2 4 3]  OutputSizes=1
  Selector4 : Selector  InputPortWidth=4  IndexOptions=Index vector (dialog)  Indices=[1 2 4 3]  OutputSizes=1
  NEh_cmd : Outport  OutDataType=sfix(16)  OutScaling=2^0
  cam_cmd : Outport  Port=2  OutDataType=sfix(16)  OutScaling=2^0
  cmd : Outport  Port=3  OutDataType=sfix(16)  OutScaling=2^0
  wires:
  Multiport Switch/1 -> cmd/1, Selector4/1
  outer cmd/1 -> Multiport Switch/4
  Bus Selector/2 -> Multiport Switch/3  "<autopilot_cmd>"
  Bus Selector/1 -> Multiport Switch/1  "<pos>"
  NEh_current/1 -> Mux1/1
  Ground/1 -> Mux1/2
  Mux1/1 -> Selector2/1
  Selector2/1 -> Multiport Switch/2
  Selector4/1 -> Demux3/1
  Demux3/1 -> NEh_cmd/1
  Demux3/2 -> cam_cmd/1
  signal_bus/1 -> Bus Selector/1
